simulink model "eqestate"  (R2015a)
settings: Solver=ode45  StartTime=0.0  StopTime=10  RelTol=1e-3
undefined symbols (not defined in the file or in its folder): deg, Equation_state_Euler, Equation_state_quat, rad, s
libraries: aerolibconvert2 x4, aerolibanim x2, aerolibtransform2 x1
settings Model: Creator=Brayan  LastModifiedBy=Brayan

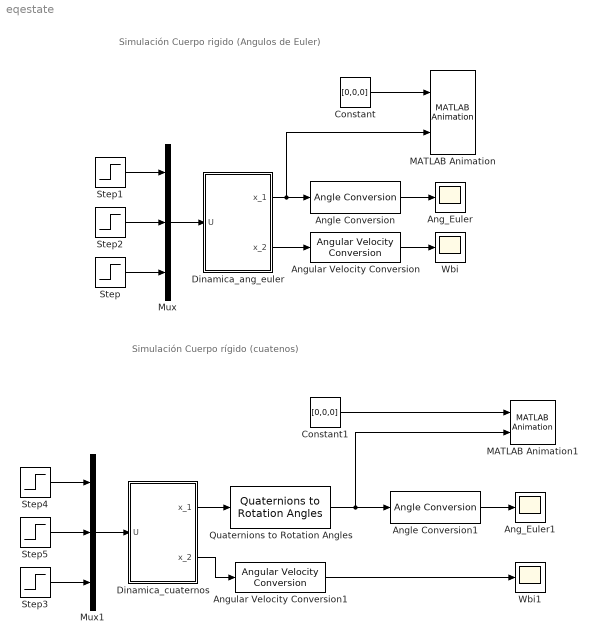
== system eqestate ==
  note: Simulación Cuerpo rígido (cuatenos)
  note: Simulación Cuerpo rigido (Angulos de Euler)
  Ang_Euler : Scope
      settings: YMin=0  YMax=1
  Ang_Euler1 : Scope
      settings: YMin=0  YMax=1  SaveName=ScopeData2
  Angle Conversion : aerolibconvert2/Angle Conversion  IU=rad  OU=deg
  Angle Conversion1 : aerolibconvert2/Angle Conversion  IU=rad  OU=deg
  Angular Velocity Conversion : aerolibconvert2/Angular Velocity Conversion  IU=deg/s  OU=rad/s
  Angular Velocity Conversion1 : aerolibconvert2/Angular Velocity Conversion  IU=deg/s  OU=rad/s
  Constant : Constant  Value=[0,0,0]
  Constant1 : Constant  Value=[0,0,0]
  Dinamica_ang_euler : Subsystem  mask{I=[1,1,1], InitialCondition=[0,0,0,0,0,0]}
      mask prompts: I "[Ix,Iy,Iz] :"; InitialCondition "Condiciones iniciales:"
      mask TypeOptions I: I/Value
      mask TypeOptions InitialCondition: Integrator1/InitialCondition
  Dinamica_cuaternos : Subsystem  mask{I=[1,1,1], InitialCondition=[1,0,0,0,0,0,0]}
      mask prompts: I "[Ix,Iy,Iz] :"; InitialCondition "Condiciones iniciales:"
      mask TypeOptions I: I/Value
      mask TypeOptions InitialCondition: Integrator1/InitialCondition
  MATLAB Animation : aerolibanim/MATLAB Animation  Tag=Matlab Animation 6 DOF  Vehicles=1  Geometries='ac3d_xyzisrgb.ac'  BoundingBoxCoordinates=[-50,50,-50,50,-50,50]  CameraOffset=[-150,-50,0]  CameraViewAngle=3  SampleTime=0.2  FigurePosition=[2,42,681,669]
  MATLAB Animation1 : aerolibanim/MATLAB Animation  Tag=Matlab Animation 6 DOF  Vehicles=1  Geometries='ac3d_xyzisrgb.ac'  BoundingBoxCoordinates=[-50,50,-50,50,-50,50]  CameraOffset=[-150,-50,0]  CameraViewAngle=3  SampleTime=0.2  FigurePosition=[2,42,681,669]
  Mux : Mux  Inputs=3
  Mux1 : Mux  Inputs=3
  Quaternions to Rotation Angles : aerolibtransform2/Quaternions to Rotation Angles  rotationOrder=ZYX
  Step : Step  Before=1  After=0  SampleTime=0
  Step{1..3,5} (4 alike) : Step  After=0  SampleTime=0
  Step4 : Step  Before=1  After=0  SampleTime=0
  Wbi : Scope
      settings: YMin=0  YMax=1
  Wbi1 : Scope
      settings: YMin=0  YMax=1  SaveName=ScopeData3
  wires:
  Step1/1 -> Mux/1
  Step2/1 -> Mux/2
  Step/1 -> Mux/3
  Dinamica_ang_euler/2("x_2 ") -> Angular Velocity Conversion/1
  Angular Velocity Conversion/1 -> Wbi/1
  Constant/1 -> MATLAB Animation/1
  Mux/1 -> Dinamica_ang_euler/1(U)
  Angle Conversion/1 -> Ang_Euler/1
  Dinamica_ang_euler/1(x_1) -> MATLAB Animation/2, Angle Conversion/1
  Step4/1 -> Mux1/1
  Step5/1 -> Mux1/2
  Step3/1 -> Mux1/3
  Dinamica_cuaternos/2("x_2 ") -> Angular Velocity Conversion1/1
  Angular Velocity Conversion1/1 -> Wbi1/1
  Quaternions to Rotation Angles/1 -> MATLAB Animation1/2, Angle Conversion1/1
  Angle Conversion1/1 -> Ang_Euler1/1
  Constant1/1 -> MATLAB Animation1/1
  Mux1/1 -> Dinamica_cuaternos/1(U)
  Dinamica_cuaternos/1(x_1) -> Quaternions to Rotation Angles/1

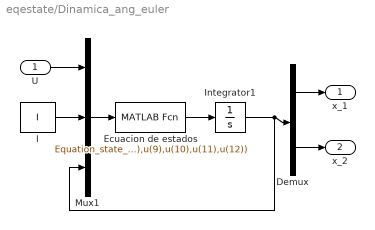
== system eqestate/Dinamica_ang_euler ==
  U : Inport
  Demux : Demux  Outputs=2
  Ecuacion de estados : MATLABFcn  MATLABFcn=Equation_state_Euler(u(1),u(2),u(3),u(4),u(5),u(6),u(7),u(8),u(9),u(10),u(11),u(12))
  I : Constant  Value=I
  Integrator1 : Integrator  InitialCondition=InitialCondition
  Mux1 : Mux  Inputs=3
  x_1 : Outport
  "x_2 " : Outport  Port=2
  wires:
  Demux/1 -> x_1/1
  Integrator1/1 -> Mux1/3, Demux/1
  Demux/2 -> "x_2 "/1
  U/1 -> Mux1/1
  Ecuacion de estados/1 -> Integrator1/1
  Mux1/1 -> Ecuacion de estados/1
  I/1 -> Mux1/2

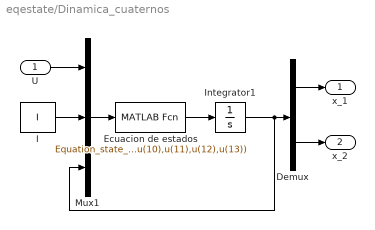
== system eqestate/Dinamica_cuaternos ==
  U : Inport
  Demux : Demux  Outputs=2
  Ecuacion de estados : MATLABFcn  MATLABFcn=Equation_state_quat(u(1),u(2),u(3),u(4),u(5),u(6),u(7),u(8),u(9),u(10),u(11),u(12),u(13))
  I : Constant  Value=I
  Integrator1 : Integrator  InitialCondition=InitialCondition
  Mux1 : Mux  Inputs=3
  x_1 : Outport
  "x_2 " : Outport  Port=2
  wires:
  Demux/1 -> x_1/1
  Integrator1/1 -> Mux1/3, Demux/1
  Demux/2 -> "x_2 "/1
  U/1 -> Mux1/1
  Ecuacion de estados/1 -> Integrator1/1
  Mux1/1 -> Ecuacion de estados/1
  I/1 -> Mux1/2
